simulink model "TopLevel"  (R2025b)
settings: Solver=VariableStepAuto  StartTime=0.0  StopTime=20  RelTol=1e-3
settings Model: Creator=mammadoo  LastModifiedBy=mammadoo

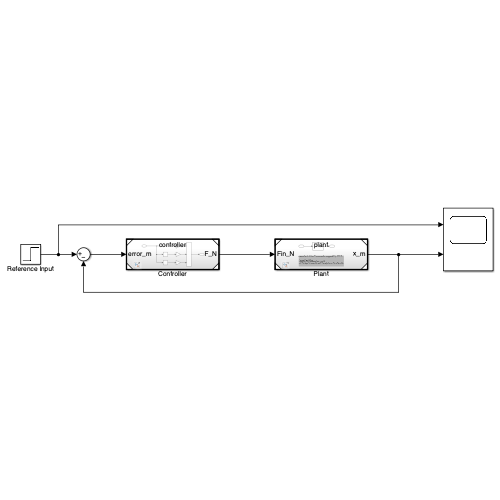
[thumbnail: Simulink's stored preview of the top-level diagram]
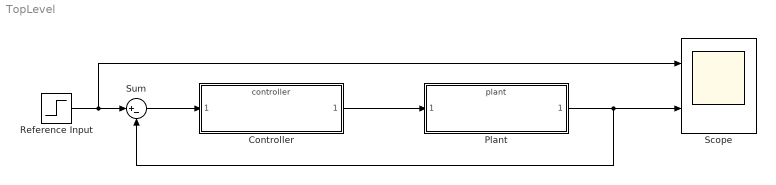
== system TopLevel ==
  Controller : ModelReference  ModelNameDialog=controller.slx  SimulationMode=Normal  ModelReferenceVersion=1.5
  Plant : ModelReference  ModelNameDialog=plant.slx  SimulationMode=Normal  ModelReferenceVersion=1.4
  Reference Input : Step  SampleTime=0
  Scope : Scope  NumInputPorts=2
      settings: ActiveDisplayYMinimum=-0.18379959452362413  ActiveDisplayYMaximum=1.6541963507126174
  Sum : Sum  Inputs=|+-
  wires:
  Controller/1 -> Plant/1
  Plant/1 -> Sum/2, Scope/2
  Sum/1 -> Controller/1
  Reference Input/1 -> Scope/1, Sum/1
